simulink model "CRH2forBenchmark_Copy"  (R2014a)
settings: Solver=ode3  StartTime=0.0  StopTime=1  FixedStep=1e-5  RelTol=1e-3
PostLoadFcn:
  | , if any(exist('dsrtsu_mdlpostloadfcn', 'file') == [2, 3, 6]), try dsrtsu_mdlpostloadfcn('Execute', bdroot); catch fprintf('Error in PostLoadFcn (dsrtsu_mdlpostloadfcn) for model "%s":\n %s\n', bdroot, lasterr); end, end,
values from neighbouring files (symbols this model uses):
  Cd = 0.016    [CRH2forBenchmark.mat]
  Lm = 0.032848    [CRH2forBenchmark.mat]
  Ln = 0.002    [CRH2forBenchmark.mat]
  Lr = 0.034142    [CRH2forBenchmark.mat]
  Ls = 0.0342654    [CRH2forBenchmark.mat]
  np = 2    [CRH2forBenchmark.mat]
  Rd = 6000    [CRH2forBenchmark.mat]
  Rn = 0.2    [CRH2forBenchmark.mat]
  Rr = 0.146    [CRH2forBenchmark.mat]
  Rs = 0.144    [CRH2forBenchmark.mat]
  ts = 1e-05    [CRH2forBenchmark.mat]
undefined symbols (not defined in the file): J, KIM, KIT, KPM, KPT, phir, Ts, Vge
libraries: simulink x20
(part 4 of 5)

== system CRH2forBenchmark_Copy/ConverterF/Rectifier/RecSubF/SABF ==
  SA : Inport
  SB : Inport  Port=2
  SABF_sfcn : S-Function  FunctionName=SABF_sf  SFunctionModules=""  EnableBusSupport=off  mask{rtw_sf_name=SABF_sf, showVar=off}
      mask prompts: rtw_sf_name "Simulink:masks:GenSFuncName_MP"; showVar "Simulink:masks:GenSFuncShowModuleList_MP"
      mask help: Simulink:masks:GenSFuncDesc_MD
      mask init: same as CRH2forBenchmark_Copy/DCU1/DCU1_sfcn
      settings: CopyFcn=|
      | if ~strcmp(get_param(gcb,'Linkstatus'),'none') && ...
      | ~strcmp(get_param(gcb,'Linkstatus'),'implicit')
      |   set_param(gcb,'LinkStatus','none');
      | end
      mask Help: eval('feval(''rtwprivate'',''rtwhelpview'',''rtw_sfcn_block'')');
      mask Display:
      | port_label('input',1,'SA');
      | port_label('input',2,'SB');
      | port_label('output',1,'P');
      | port_label('output',2,'O');
      | port_label('output',3,'N');
  __InputSSForSFun__ : Subsystem
  __OutputSSForSFun__ : Subsystem
  P : Outport
  O : Outport  Port=2
  N : Outport  Port=3
  wires:
  SA/1 -> __InputSSForSFun__/1(SA)
  SB/1 -> __InputSSForSFun__/2(SB)
  __InputSSForSFun__/1(__UniqueOutportName__1__) -> SABF_sfcn/1
  __InputSSForSFun__/2(__UniqueOutportName__2__) -> SABF_sfcn/2
  SABF_sfcn/1 -> __OutputSSForSFun__/1(__UniqueInportName__1__)
  SABF_sfcn/2 -> __OutputSSForSFun__/2(__UniqueInportName__2__)
  SABF_sfcn/3 -> __OutputSSForSFun__/3(__UniqueInportName__3__)
  __OutputSSForSFun__/1(P) -> P/1
  __OutputSSForSFun__/2(O) -> O/1
  __OutputSSForSFun__/3(N) -> N/1

== system CRH2forBenchmark_Copy/ConverterF/Rectifier/RecSubF/SAF ==
  Ta1 : Inport
  Ta2 : Inport  Port=2
  Ta3 : Inport  Port=3
  Ta4 : Inport  Port=4
  In : Inport  Port=5
  SAF_sfcn : S-Function  FunctionName=SAF_sf  SFunctionModules=""  EnableBusSupport=off  mask{rtw_sf_name=SAF_sf, showVar=off}
      mask prompts: rtw_sf_name "Simulink:masks:GenSFuncName_MP"; showVar "Simulink:masks:GenSFuncShowModuleList_MP"
      mask help: Simulink:masks:GenSFuncDesc_MD
      mask init: same as CRH2forBenchmark_Copy/DCU1/DCU1_sfcn
      settings: CopyFcn=|
      | if ~strcmp(get_param(gcb,'Linkstatus'),'none') && ...
      | ~strcmp(get_param(gcb,'Linkstatus'),'implicit')
      |   set_param(gcb,'LinkStatus','none');
      | end
      mask Help: eval('feval(''rtwprivate'',''rtwhelpview'',''rtw_sfcn_block'')');
      mask Display:
      | port_label('input',1,'Ta1');
      | port_label('input',2,'Ta2');
      | port_label('input',3,'Ta3');
      | port_label('input',4,'Ta4');
      | port_label('input',5,'In');
      | port_label('output',1,'SA');
  __InputSSForSFun__ : Subsystem
  __OutputSSForSFun__ : Subsystem
  SA : Outport
  wires:
  Ta1/1 -> __InputSSForSFun__/1(Ta1)
  Ta2/1 -> __InputSSForSFun__/2(Ta2)
  Ta3/1 -> __InputSSForSFun__/3(Ta3)
  Ta4/1 -> __InputSSForSFun__/4(Ta4)
  In/1 -> __InputSSForSFun__/5(In)
  __InputSSForSFun__/1(__UniqueOutportName__1__) -> SAF_sfcn/1
  __InputSSForSFun__/2(__UniqueOutportName__2__) -> SAF_sfcn/2
  __InputSSForSFun__/3(__UniqueOutportName__3__) -> SAF_sfcn/3
  __InputSSForSFun__/4(__UniqueOutportName__4__) -> SAF_sfcn/4
  __InputSSForSFun__/5(__UniqueOutportName__5__) -> SAF_sfcn/5
  SAF_sfcn/1 -> __OutputSSForSFun__/1(__UniqueInportName__1__)
  __OutputSSForSFun__/1(SA) -> SA/1

== system CRH2forBenchmark_Copy/ConverterF/Rectifier/RecSubF/SBF ==
  Tb1 : Inport
  Tb2 : Inport  Port=2
  Tb3 : Inport  Port=3
  Tb4 : Inport  Port=4
  In : Inport  Port=5
  SBF_sfcn : S-Function  FunctionName=SBF_sf  SFunctionModules=""  EnableBusSupport=off  mask{rtw_sf_name=SBF_sf, showVar=off}
      mask prompts: rtw_sf_name "Simulink:masks:GenSFuncName_MP"; showVar "Simulink:masks:GenSFuncShowModuleList_MP"
      mask help: Simulink:masks:GenSFuncDesc_MD
      mask init: same as CRH2forBenchmark_Copy/DCU1/DCU1_sfcn
      settings: CopyFcn=|
      | if ~strcmp(get_param(gcb,'Linkstatus'),'none') && ...
      | ~strcmp(get_param(gcb,'Linkstatus'),'implicit')
      |   set_param(gcb,'LinkStatus','none');
      | end
      mask Help: eval('feval(''rtwprivate'',''rtwhelpview'',''rtw_sfcn_block'')');
      mask Display:
      | port_label('input',1,'Tb1');
      | port_label('input',2,'Tb2');
      | port_label('input',3,'Tb3');
      | port_label('input',4,'Tb4');
      | port_label('input',5,'In');
      | port_label('output',1,'SB');
  __InputSSForSFun__ : Subsystem
  __OutputSSForSFun__ : Subsystem
  SB : Outport
  wires:
  Tb1/1 -> __InputSSForSFun__/1(Tb1)
  Tb2/1 -> __InputSSForSFun__/2(Tb2)
  Tb3/1 -> __InputSSForSFun__/3(Tb3)
  Tb4/1 -> __InputSSForSFun__/4(Tb4)
  In/1 -> __InputSSForSFun__/5(In)
  __InputSSForSFun__/1(__UniqueOutportName__1__) -> SBF_sfcn/1
  __InputSSForSFun__/2(__UniqueOutportName__2__) -> SBF_sfcn/2
  __InputSSForSFun__/3(__UniqueOutportName__3__) -> SBF_sfcn/3
  __InputSSForSFun__/4(__UniqueOutportName__4__) -> SBF_sfcn/4
  __InputSSForSFun__/5(__UniqueOutportName__5__) -> SBF_sfcn/5
  SBF_sfcn/1 -> __OutputSSForSFun__/1(__UniqueInportName__1__)
  __OutputSSForSFun__/1(SB) -> SB/1

== system CRH2forBenchmark_Copy/ConverterN/Rectifier/RecSubN/RecSubSubN ==
  In1 : Inport
  In2 : Inport  Port=2
  In3 : Inport  Port=3
  In4 : Inport  Port=4
  In5 : Inport  Port=5
  In6 : Inport  Port=6
  RecSubSubN_sfcn : S-Function  FunctionName=RecSubSubN_sf  SFunctionModules=""  EnableBusSupport=off  mask{rtw_sf_name=RecSubSubN_sf, showVar=off}
      mask prompts: rtw_sf_name "Simulink:masks:GenSFuncName_MP"; showVar "Simulink:masks:GenSFuncShowModuleList_MP"
      mask help: Simulink:masks:GenSFuncDesc_MD
      mask init: same as CRH2forBenchmark_Copy/DCU1/DCU1_sfcn
      settings: CopyFcn=|
      | if ~strcmp(get_param(gcb,'Linkstatus'),'none') && ...
      | ~strcmp(get_param(gcb,'Linkstatus'),'implicit')
      |   set_param(gcb,'LinkStatus','none');
      | end
      mask Help: eval('feval(''rtwprivate'',''rtwhelpview'',''rtw_sfcn_block'')');
      mask Display:
      | port_label('input',1,'In1');
      | port_label('input',2,'In2');
      | port_label('input',3,'In3');
      | port_label('input',4,'In4');
      | port_label('input',5,'In5');
      | port_label('input',6,'In6');
      | port_label('output',1,'Out1');
      | port_label('output',2,'Out2');
  __InputSSForSFun__ : Subsystem
  __OutputSSForSFun__ : Subsystem
  Out1 : Outport
  Out2 : Outport  Port=2
  wires:
  In1/1 -> __InputSSForSFun__/1(In1)
  In2/1 -> __InputSSForSFun__/2(In2)
  In3/1 -> __InputSSForSFun__/3(In3)
  In4/1 -> __InputSSForSFun__/4(In4)
  In5/1 -> __InputSSForSFun__/5(In5)
  In6/1 -> __InputSSForSFun__/6(In6)
  __InputSSForSFun__/1(__UniqueOutportName__1__) -> RecSubSubN_sfcn/1
  __InputSSForSFun__/2(__UniqueOutportName__2__) -> RecSubSubN_sfcn/2
  __InputSSForSFun__/3(__UniqueOutportName__3__) -> RecSubSubN_sfcn/3
  __InputSSForSFun__/4(__UniqueOutportName__4__) -> RecSubSubN_sfcn/4
  __InputSSForSFun__/5(__UniqueOutportName__5__) -> RecSubSubN_sfcn/5
  __InputSSForSFun__/6(__UniqueOutportName__6__) -> RecSubSubN_sfcn/6
  RecSubSubN_sfcn/1 -> __OutputSSForSFun__/1(__UniqueInportName__1__)
  RecSubSubN_sfcn/2 -> __OutputSSForSFun__/2(__UniqueInportName__2__)
  __OutputSSForSFun__/1(Out1) -> Out1/1
  __OutputSSForSFun__/2(Out2) -> Out2/1

== system CRH2forBenchmark_Copy/ConverterN/Rectifier/RecSubN/SABN ==
  SA : Inport
  SB : Inport  Port=2
  SABN_sfcn : S-Function  FunctionName=SABN_sf  SFunctionModules=""  EnableBusSupport=off  mask{rtw_sf_name=SABN_sf, showVar=off}
      mask prompts: rtw_sf_name "Simulink:masks:GenSFuncName_MP"; showVar "Simulink:masks:GenSFuncShowModuleList_MP"
      mask help: Simulink:masks:GenSFuncDesc_MD
      mask init: same as CRH2forBenchmark_Copy/DCU1/DCU1_sfcn
      settings: CopyFcn=|
      | if ~strcmp(get_param(gcb,'Linkstatus'),'none') && ...
      | ~strcmp(get_param(gcb,'Linkstatus'),'implicit')
      |   set_param(gcb,'LinkStatus','none');
      | end
      mask Help: eval('feval(''rtwprivate'',''rtwhelpview'',''rtw_sfcn_block'')');
      mask Display:
      | port_label('input',1,'SA');
      | port_label('input',2,'SB');
      | port_label('output',1,'P');
      | port_label('output',2,'O');
      | port_label('output',3,'N');
  __InputSSForSFun__ : Subsystem
  __OutputSSForSFun__ : Subsystem
  P : Outport
  O : Outport  Port=2
  N : Outport  Port=3
  wires:
  SA/1 -> __InputSSForSFun__/1(SA)
  SB/1 -> __InputSSForSFun__/2(SB)
  __InputSSForSFun__/1(__UniqueOutportName__1__) -> SABN_sfcn/1
  __InputSSForSFun__/2(__UniqueOutportName__2__) -> SABN_sfcn/2
  SABN_sfcn/1 -> __OutputSSForSFun__/1(__UniqueInportName__1__)
  SABN_sfcn/2 -> __OutputSSForSFun__/2(__UniqueInportName__2__)
  SABN_sfcn/3 -> __OutputSSForSFun__/3(__UniqueInportName__3__)
  __OutputSSForSFun__/1(P) -> P/1
  __OutputSSForSFun__/2(O) -> O/1
  __OutputSSForSFun__/3(N) -> N/1

== system CRH2forBenchmark_Copy/ConverterN/Rectifier/RecSubN/SAN ==
  Ta1 : Inport
  Ta2 : Inport  Port=2
  Ta3 : Inport  Port=3
  Ta4 : Inport  Port=4
  In : Inport  Port=5
  SAN_sfcn : S-Function  FunctionName=SAN_sf  SFunctionModules=""  EnableBusSupport=off  mask{rtw_sf_name=SAN_sf, showVar=off}
      mask prompts: rtw_sf_name "Simulink:masks:GenSFuncName_MP"; showVar "Simulink:masks:GenSFuncShowModuleList_MP"
      mask help: Simulink:masks:GenSFuncDesc_MD
      mask init: same as CRH2forBenchmark_Copy/DCU1/DCU1_sfcn
      settings: CopyFcn=|
      | if ~strcmp(get_param(gcb,'Linkstatus'),'none') && ...
      | ~strcmp(get_param(gcb,'Linkstatus'),'implicit')
      |   set_param(gcb,'LinkStatus','none');
      | end
      mask Help: eval('feval(''rtwprivate'',''rtwhelpview'',''rtw_sfcn_block'')');
      mask Display:
      | port_label('input',1,'Ta1');
      | port_label('input',2,'Ta2');
      | port_label('input',3,'Ta3');
      | port_label('input',4,'Ta4');
      | port_label('input',5,'In');
      | port_label('output',1,'SA');
  __InputSSForSFun__ : Subsystem
  __OutputSSForSFun__ : Subsystem
  SA : Outport
  wires:
  Ta1/1 -> __InputSSForSFun__/1(Ta1)
  Ta2/1 -> __InputSSForSFun__/2(Ta2)
  Ta3/1 -> __InputSSForSFun__/3(Ta3)
  Ta4/1 -> __InputSSForSFun__/4(Ta4)
  In/1 -> __InputSSForSFun__/5(In)
  __InputSSForSFun__/1(__UniqueOutportName__1__) -> SAN_sfcn/1
  __InputSSForSFun__/2(__UniqueOutportName__2__) -> SAN_sfcn/2
  __InputSSForSFun__/3(__UniqueOutportName__3__) -> SAN_sfcn/3
  __InputSSForSFun__/4(__UniqueOutportName__4__) -> SAN_sfcn/4
  __InputSSForSFun__/5(__UniqueOutportName__5__) -> SAN_sfcn/5
  SAN_sfcn/1 -> __OutputSSForSFun__/1(__UniqueInportName__1__)
  __OutputSSForSFun__/1(SA) -> SA/1

== system CRH2forBenchmark_Copy/ConverterN/Rectifier/RecSubN/SBN ==
  Tb1 : Inport
  Tb2 : Inport  Port=2
  Tb3 : Inport  Port=3
  Tb4 : Inport  Port=4
  In : Inport  Port=5
  SBN_sfcn : S-Function  FunctionName=SBN_sf  SFunctionModules=""  EnableBusSupport=off  mask{rtw_sf_name=SBN_sf, showVar=off}
      mask prompts: rtw_sf_name "Simulink:masks:GenSFuncName_MP"; showVar "Simulink:masks:GenSFuncShowModuleList_MP"
      mask help: Simulink:masks:GenSFuncDesc_MD
      mask init: same as CRH2forBenchmark_Copy/DCU1/DCU1_sfcn
      settings: CopyFcn=|
      | if ~strcmp(get_param(gcb,'Linkstatus'),'none') && ...
      | ~strcmp(get_param(gcb,'Linkstatus'),'implicit')
      |   set_param(gcb,'LinkStatus','none');
      | end
      mask Help: eval('feval(''rtwprivate'',''rtwhelpview'',''rtw_sfcn_block'')');
      mask Display:
      | port_label('input',1,'Tb1');
      | port_label('input',2,'Tb2');
      | port_label('input',3,'Tb3');
      | port_label('input',4,'Tb4');
      | port_label('input',5,'In');
      | port_label('output',1,'SB');
  __InputSSForSFun__ : Subsystem
  __OutputSSForSFun__ : Subsystem
  SB : Outport
  wires:
  Tb1/1 -> __InputSSForSFun__/1(Tb1)
  Tb2/1 -> __InputSSForSFun__/2(Tb2)
  Tb3/1 -> __InputSSForSFun__/3(Tb3)
  Tb4/1 -> __InputSSForSFun__/4(Tb4)
  In/1 -> __InputSSForSFun__/5(In)
  __InputSSForSFun__/1(__UniqueOutportName__1__) -> SBN_sfcn/1
  __InputSSForSFun__/2(__UniqueOutportName__2__) -> SBN_sfcn/2
  __InputSSForSFun__/3(__UniqueOutportName__3__) -> SBN_sfcn/3
  __InputSSForSFun__/4(__UniqueOutportName__4__) -> SBN_sfcn/4
  __InputSSForSFun__/5(__UniqueOutportName__5__) -> SBN_sfcn/5
  SBN_sfcn/1 -> __OutputSSForSFun__/1(__UniqueInportName__1__)
  __OutputSSForSFun__/1(SB) -> SB/1

== system CRH2forBenchmark_Copy/Machine model/Normal ModelF/MeasurementF/__InputSSForSFun__ ==
  isα : Inport
  isβ : Inport  Port=2
  irα : Inport  Port=3
  irβ : Inport  Port=4
  TL : Inport  Port=5
  __UniqueOutportName__1__ : Outport
  __UniqueOutportName__2__ : Outport  Port=2
  __UniqueOutportName__3__ : Outport  Port=3
  __UniqueOutportName__4__ : Outport  Port=4
  __UniqueOutportName__5__ : Outport  Port=5
  wires:
  isα/1 -> __UniqueOutportName__1__/1
  isβ/1 -> __UniqueOutportName__2__/1
  irα/1 -> __UniqueOutportName__3__/1
  irβ/1 -> __UniqueOutportName__4__/1
  TL/1 -> __UniqueOutportName__5__/1

== system CRH2forBenchmark_Copy/Machine model/Normal ModelF/MeasurementF/__OutputSSForSFun__ ==
  __UniqueInportName__1__ : Inport
  __UniqueInportName__2__ : Inport  Port=2
  __UniqueInportName__3__ : Inport  Port=3
  Te : Outport
  ω : Outport  Port=2
  Isabc : Outport  Port=3
  wires:
  __UniqueInportName__1__/1 -> Te/1
  __UniqueInportName__2__/1 -> ω/1
  __UniqueInportName__3__/1 -> Isabc/1

== system CRH2forBenchmark_Copy/Machine model/Normal ModelF/MotorSubsystem1F/MotorSubsystem1FSub ==
  note: 1/(Ls*Lr-Lm*Lm)
  ψrβ : Inport
  Usβ : Inport  Port=2
  Add : Sum  Inputs=+-
  Add1 : Sum  Inputs=-+
  Gain : Gain  Gain=Lm
  Gain1 : Gain  Gain=Lr
  Gain2 : Gain  Gain=1/(Ls*Lr-Lm*Lm)
  Gain3 : Gain  Gain=Rs
  Integrator : Integrator
  isβ : Outport
  ψsβ : Outport  Port=2
  wires:
  Gain3/1 -> Add1/1
  ψrβ/1 -> Gain/1
  Gain2/1 -> isβ/1, Gain3/1
  Gain/1 -> Add/2
  Usβ/1 -> Add1/2
  Gain1/1 -> Add/1
  Add1/1 -> Integrator/1
  Add/1 -> Gain2/1
  Integrator/1 -> ψsβ/1, Gain1/1

== system CRH2forBenchmark_Copy/Machine model/Normal ModelF/MotorSubsystem2F/MotorSubsystem2FSub ==
  ψsα : Inport
  ψrβ : Inport  Port=2
  ω : Inport  Port=3
  1/(Ls*Lr-Lm*Lm) : Gain  Gain=1/(Ls*Lr-Lm*Lm)
  Add : Sum  Inputs=+-
  Add1 : Sum  Inputs=--
  Gain : Gain  Gain=Lm
  Gain1 : Gain  Gain=Ls
  Gain3 : Gain  Gain=Rr
  Integrator : Integrator
  Product : Product
  irα : Outport
  ψrα : Outport  Port=2
  wires:
  Add1/1 -> Integrator/1
  ω/1 -> Product/1
  Product/1 -> Add1/2
  ψrβ/1 -> Product/2
  Gain/1 -> Add/2
  Integrator/1 -> ψrα/1, Gain1/1
  1/(Ls*Lr-Lm*Lm)/1 -> irα/1, Gain3/1
  Add/1 -> 1/(Ls*Lr-Lm*Lm)/1
  ψsα/1 -> Gain/1
  Gain1/1 -> Add/1
  Gain3/1 -> Add1/1

== system CRH2forBenchmark_Copy/Machine model/Normal ModelF/MotorSubsystem3F/MotorSubsystem3FSub ==
  ψsβ : Inport
  ψrα : Inport  Port=2
  ω : Inport  Port=3
  1/(Ls*Lr-Lm*Lm) : Gain  Gain=1/(Ls*Lr-Lm*Lm)
  Add : Sum  Inputs=+-
  Add1 : Sum  Inputs=-+
  Gain : Gain  Gain=Lm
  Gain1 : Gain  Gain=Ls
  Gain3 : Gain  Gain=Rr
  Integrator : Integrator
  Product : Product
  irβ : Outport
  ψrβ : Outport  Port=2
  wires:
  Add1/1 -> Integrator/1
  Add/1 -> 1/(Ls*Lr-Lm*Lm)/1
  ψrα/1 -> Product/2
  Gain3/1 -> Add1/1
  1/(Ls*Lr-Lm*Lm)/1 -> irβ/1, Gain3/1
  ψsβ/1 -> Gain/1
  Gain1/1 -> Add/1
  Gain/1 -> Add/2
  ω/1 -> Product/1
  Product/1 -> Add1/2
  Integrator/1 -> ψrβ/1, Gain1/1

== system CRH2forBenchmark_Copy/Machine model/Normal ModelF/MotorSubsystemF/MotorSubsystemFSub ==
  note: 1/(Ls*Lr-Lm*Lm)
  ψrα : Inport
  Usα : Inport  Port=2
  Add : Sum  Inputs=+-
  Add1 : Sum  Inputs=-+
  Gain : Gain  Gain=Lm
  Gain1 : Gain  Gain=Lr
  Gain2 : Gain  Gain=1/(Ls*Lr-Lm*Lm)
  Gain3 : Gain  Gain=Rs
  Integrator : Integrator
  isα : Outport
  ψsα : Outport  Port=2
  wires:
  Add1/1 -> Integrator/1
  Add/1 -> Gain2/1
  Integrator/1 -> ψsα/1, Gain1/1
  Gain2/1 -> isα/1, Gain3/1
  Usα/1 -> Add1/2
  Gain3/1 -> Add1/1
  Gain1/1 -> Add/1
  ψrα/1 -> Gain/1
  Gain/1 -> Add/2

== system CRH2forBenchmark_Copy/Machine model/Normal ModelF/r2sF/__InputSSForSFun__ ==
  Ua : Inport
  Ub : Inport  Port=2
  Uc : Inport  Port=3
  __UniqueOutportName__1__ : Outport
  __UniqueOutportName__2__ : Outport  Port=2
  __UniqueOutportName__3__ : Outport  Port=3
  wires:
  Ua/1 -> __UniqueOutportName__1__/1
  Ub/1 -> __UniqueOutportName__2__/1
  Uc/1 -> __UniqueOutportName__3__/1

== system CRH2forBenchmark_Copy/Machine model/Normal ModelF/r2sF/__OutputSSForSFun__ ==
  __UniqueInportName__1__ : Inport
  __UniqueInportName__2__ : Inport  Port=2
  Usα : Outport
  Usβ : Outport  Port=2
  wires:
  __UniqueInportName__1__/1 -> Usα/1
  __UniqueInportName__2__/1 -> Usβ/1

== system CRH2forBenchmark_Copy/Machine model1/Normal ModelN/MeasurementN/__InputSSForSFun__ ==
  isα : Inport
  isβ : Inport  Port=2
  irα : Inport  Port=3
  irβ : Inport  Port=4
  TL : Inport  Port=5
  __UniqueOutportName__1__ : Outport
  __UniqueOutportName__2__ : Outport  Port=2
  __UniqueOutportName__3__ : Outport  Port=3
  __UniqueOutportName__4__ : Outport  Port=4
  __UniqueOutportName__5__ : Outport  Port=5
  wires:
  isα/1 -> __UniqueOutportName__1__/1
  isβ/1 -> __UniqueOutportName__2__/1
  irα/1 -> __UniqueOutportName__3__/1
  irβ/1 -> __UniqueOutportName__4__/1
  TL/1 -> __UniqueOutportName__5__/1

== system CRH2forBenchmark_Copy/Machine model1/Normal ModelN/MeasurementN/__OutputSSForSFun__ ==
  __UniqueInportName__1__ : Inport
  __UniqueInportName__2__ : Inport  Port=2
  __UniqueInportName__3__ : Inport  Port=3
  Te : Outport
  ω : Outport  Port=2
  Isabc : Outport  Port=3
  wires:
  __UniqueInportName__1__/1 -> Te/1
  __UniqueInportName__2__/1 -> ω/1
  __UniqueInportName__3__/1 -> Isabc/1

== system CRH2forBenchmark_Copy/Machine model1/Normal ModelN/MotorSubsystem1N/MotorSubsystem1NSub ==
  note: 1/(Ls*Lr-Lm*Lm)
  ψrβ : Inport
  Usβ : Inport  Port=2
  Add : Sum  Inputs=+-
  Add1 : Sum  Inputs=-+
  Gain : Gain  Gain=Lm
  Gain1 : Gain  Gain=Lr
  Gain2 : Gain  Gain=1/(Ls*Lr-Lm*Lm)
  Gain3 : Gain  Gain=Rs
  Integrator : Integrator
  isβ : Outport
  ψsβ : Outport  Port=2
  wires:
  Gain3/1 -> Add1/1
  ψrβ/1 -> Gain/1
  Gain2/1 -> isβ/1, Gain3/1
  Gain/1 -> Add/2
  Usβ/1 -> Add1/2
  Gain1/1 -> Add/1
  Add1/1 -> Integrator/1
  Add/1 -> Gain2/1
  Integrator/1 -> ψsβ/1, Gain1/1

== system CRH2forBenchmark_Copy/Machine model1/Normal ModelN/MotorSubsystem2N/MotorSubsystem2NSub ==
  ψsα : Inport
  ψrβ : Inport  Port=2
  ω : Inport  Port=3
  1/(Ls*Lr-Lm*Lm) : Gain  Gain=1/(Ls*Lr-Lm*Lm)
  Add : Sum  Inputs=+-
  Add1 : Sum  Inputs=--
  Gain : Gain  Gain=Lm
  Gain1 : Gain  Gain=Ls
  Gain3 : Gain  Gain=Rr
  Integrator : Integrator
  Product : Product
  irα : Outport
  ψrα : Outport  Port=2
  wires:
  Add1/1 -> Integrator/1
  ω/1 -> Product/1
  Product/1 -> Add1/2
  ψrβ/1 -> Product/2
  Gain/1 -> Add/2
  Integrator/1 -> ψrα/1, Gain1/1
  1/(Ls*Lr-Lm*Lm)/1 -> irα/1, Gain3/1
  Add/1 -> 1/(Ls*Lr-Lm*Lm)/1
  ψsα/1 -> Gain/1
  Gain1/1 -> Add/1
  Gain3/1 -> Add1/1

== system CRH2forBenchmark_Copy/Machine model1/Normal ModelN/MotorSubsystem3N/MotorSubsystem3NSub ==
  ψsβ : Inport
  ψrα : Inport  Port=2
  ω : Inport  Port=3
  1/(Ls*Lr-Lm*Lm) : Gain  Gain=1/(Ls*Lr-Lm*Lm)
  Add : Sum  Inputs=+-
  Add1 : Sum  Inputs=-+
  Gain : Gain  Gain=Lm
  Gain1 : Gain  Gain=Ls
  Gain3 : Gain  Gain=Rr
  Integrator : Integrator
  Product : Product
  irβ : Outport
  ψrβ : Outport  Port=2
  wires:
  Add1/1 -> Integrator/1
  Add/1 -> 1/(Ls*Lr-Lm*Lm)/1
  ψrα/1 -> Product/2
  Gain3/1 -> Add1/1
  1/(Ls*Lr-Lm*Lm)/1 -> irβ/1, Gain3/1
  ψsβ/1 -> Gain/1
  Gain1/1 -> Add/1
  Gain/1 -> Add/2
  ω/1 -> Product/1
  Product/1 -> Add1/2
  Integrator/1 -> ψrβ/1, Gain1/1

== system CRH2forBenchmark_Copy/Machine model1/Normal ModelN/MotorSubsystemN/MotorSubsystemNSub ==
  note: 1/(Ls*Lr-Lm*Lm)
  ψrα : Inport
  Usα : Inport  Port=2
  Add : Sum  Inputs=+-
  Add1 : Sum  Inputs=-+
  Gain : Gain  Gain=Lm
  Gain1 : Gain  Gain=Lr
  Gain2 : Gain  Gain=1/(Ls*Lr-Lm*Lm)
  Gain3 : Gain  Gain=Rs
  Integrator : Integrator
  isα : Outport
  ψsα : Outport  Port=2
  wires:
  Add1/1 -> Integrator/1
  Add/1 -> Gain2/1
  Integrator/1 -> ψsα/1, Gain1/1
  Gain2/1 -> isα/1, Gain3/1
  Usα/1 -> Add1/2
  Gain3/1 -> Add1/1
  Gain1/1 -> Add/1
  ψrα/1 -> Gain/1
  Gain/1 -> Add/2

== system CRH2forBenchmark_Copy/Machine model1/Normal ModelN/r2sN/__InputSSForSFun__ ==
  Ua : Inport
  Ub : Inport  Port=2
  Uc : Inport  Port=3
  __UniqueOutportName__1__ : Outport
  __UniqueOutportName__2__ : Outport  Port=2
  __UniqueOutportName__3__ : Outport  Port=3
  wires:
  Ua/1 -> __UniqueOutportName__1__/1
  Ub/1 -> __UniqueOutportName__2__/1
  Uc/1 -> __UniqueOutportName__3__/1

== system CRH2forBenchmark_Copy/Machine model1/Normal ModelN/r2sN/__OutputSSForSFun__ ==
  __UniqueInportName__1__ : Inport
  __UniqueInportName__2__ : Inport  Port=2
  Usα : Outport
  Usβ : Outport  Port=2
  wires:
  __UniqueInportName__1__/1 -> Usα/1
  __UniqueInportName__2__/1 -> Usβ/1

== system CRH2forBenchmark_Copy/Benchmark/CFI1/Subsystem2/Subsystem/Fault-States ==
  In1 : Inport
  Constant1 : Constant  Value=ContantofPowerDevice(1,1)
  Constant2 : Constant  Value=ContantofPowerDevice(2,1)
  Constant3 : Constant  Value=ContantofPowerDevice(3,1)
  Multiport Switch1 : MultiPortSwitch  DiagnosticForDefault=None
  Out1 : Outport
  wires:
  Constant2/1 -> Multiport Switch1/3
  Constant3/1 -> Multiport Switch1/4
  Constant1/1 -> Multiport Switch1/2
  In1/1 -> Multiport Switch1/1
  Multiport Switch1/1 -> Out1/1

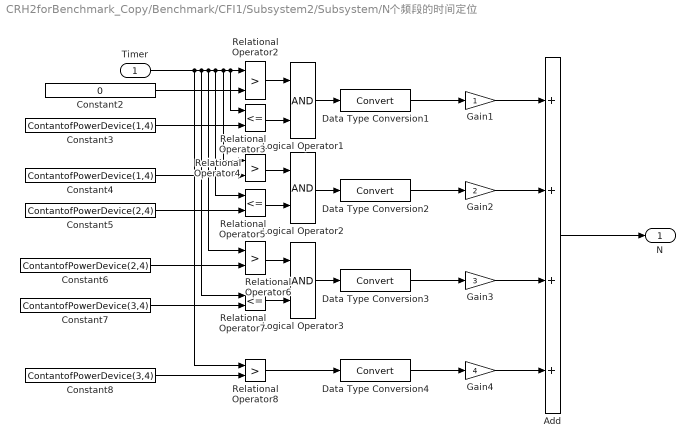
== system CRH2forBenchmark_Copy/Benchmark/CFI1/Subsystem2/Subsystem/N个频段的时间定位 ==
  Timer : Inport
  Add : Sum  Inputs=++++
  Constant2 : Constant  Value=0
  Constant3 : Constant  Value=ContantofPowerDevice(1,4)
  Constant4 : Constant  Value=ContantofPowerDevice(1,4)
  Constant5 : Constant  Value=ContantofPowerDevice(2,4)
  Constant6 : Constant  Value=ContantofPowerDevice(2,4)
  Constant7 : Constant  Value=ContantofPowerDevice(3,4)
  Constant8 : Constant  Value=ContantofPowerDevice(3,4)
  Data Type Conversion{1..4} (4 alike) : DataTypeConversion
  Gain1 : Gain
  Gain2 : Gain  Gain=2
  Gain3 : Gain  Gain=3
  Gain4 : Gain  Gain=4
  Logical Operator1 : Logic  AllPortsSameDT=off  OutDataTypeStr=boolean
  Logical Operator2 : Logic  AllPortsSameDT=off  OutDataTypeStr=boolean
  Logical Operator3 : Logic  AllPortsSameDT=off  OutDataTypeStr=boolean
  Relational Operator{2,4,6,8} (4 alike) : RelationalOperator  Operator=>  OutDataTypeStr=boolean
  Relational Operator3 : RelationalOperator  Operator=<=  OutDataTypeStr=boolean
  Relational Operator5 : RelationalOperator  Operator=<=  OutDataTypeStr=boolean
  Relational Operator7 : RelationalOperator  Operator=<=  OutDataTypeStr=boolean
  N : Outport
  wires:
  Gain4/1 -> Add/4
  Gain3/1 -> Add/3
  Gain2/1 -> Add/2
  Gain1/1 -> Add/1
  Add/1 -> N/1
  Constant8/1 -> Relational Operator8/2
  Constant7/1 -> Relational Operator7/2
  Constant6/1 -> Relational Operator6/2
  Constant5/1 -> Relational Operator5/2
  Constant4/1 -> Relational Operator4/2
  Constant3/1 -> Relational Operator3/2
  Constant2/1 -> Relational Operator2/2
  Timer/1 -> Relational Operator2/1, Relational Operator3/1, Relational Operator4/1, Relational Operator5/1, Relational Operator6/1, Relational Operator7/1, Relational Operator8/1
  Data Type Conversion4/1 -> Gain4/1
  Relational Operator8/1 -> Data Type Conversion4/1
  Data Type Conversion3/1 -> Gain3/1
  Logical Operator3/1 -> Data Type Conversion3/1
  Data Type Conversion2/1 -> Gain2/1
  Logical Operator2/1 -> Data Type Conversion2/1
  Data Type Conversion1/1 -> Gain1/1
  Logical Operator1/1 -> Data Type Conversion1/1
  Relational Operator7/1 -> Logical Operator3/2
  Relational Operator6/1 -> Logical Operator3/1
  Relational Operator5/1 -> Logical Operator2/2
  Relational Operator4/1 -> Logical Operator2/1
  Relational Operator3/1 -> Logical Operator1/2
  Relational Operator2/1 -> Logical Operator1/1

== system CRH2forBenchmark_Copy/Benchmark/CFI1/Subsystem2/Subsystem1/__InputSSForSFun__ ==
  Nomal : Inport
  Outside Signal1 : Inport  Port=2
  __UniqueOutportName__1__ : Outport
  __UniqueOutportName__2__ : Outport  Port=2
  __UniqueOutportName__3__ : Outport  Port=3
  __UniqueOutportName__4__ : Outport  Port=4
  wires:
  [PeriodicSignalsCFI1] -> __UniqueOutportName__4__/1
  [BandLimitedWhiteNoiseCFI1] -> __UniqueOutportName__3__/1
  Outside Signal1/1 -> __UniqueOutportName__2__/1
  Nomal/1 -> __UniqueOutportName__1__/1

== system CRH2forBenchmark_Copy/Benchmark/CFI1/Subsystem2/Subsystem1/__OutputSSForSFun__ ==
  __UniqueInportName__1__ : Inport
  Out : Outport
  wires:
  __UniqueInportName__1__/1 -> Out/1

== system CRH2forBenchmark_Copy/Benchmark/CFI2/Subsystem2/Subsystem/Fault-States ==
  In1 : Inport
  Constant1 : Constant  Value=ContantofPowerDevice(1,1)
  Constant2 : Constant  Value=ContantofPowerDevice(2,1)
  Constant3 : Constant  Value=ContantofPowerDevice(3,1)
  Multiport Switch1 : MultiPortSwitch  DiagnosticForDefault=None
  Out1 : Outport
  wires:
  Constant2/1 -> Multiport Switch1/3
  Constant3/1 -> Multiport Switch1/4
  Constant1/1 -> Multiport Switch1/2
  In1/1 -> Multiport Switch1/1
  Multiport Switch1/1 -> Out1/1

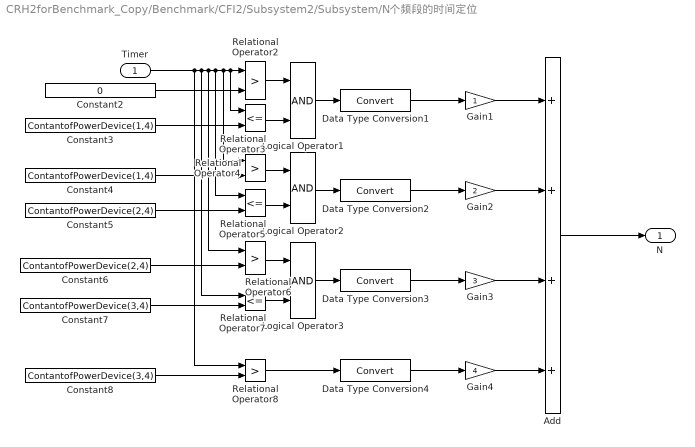
== system CRH2forBenchmark_Copy/Benchmark/CFI2/Subsystem2/Subsystem/N个频段的时间定位 ==
  Timer : Inport
  Add : Sum  Inputs=++++
  Constant2 : Constant  Value=0
  Constant3 : Constant  Value=ContantofPowerDevice(1,4)
  Constant4 : Constant  Value=ContantofPowerDevice(1,4)
  Constant5 : Constant  Value=ContantofPowerDevice(2,4)
  Constant6 : Constant  Value=ContantofPowerDevice(2,4)
  Constant7 : Constant  Value=ContantofPowerDevice(3,4)
  Constant8 : Constant  Value=ContantofPowerDevice(3,4)
  Data Type Conversion{1..4} (4 alike) : DataTypeConversion
  Gain1 : Gain
  Gain2 : Gain  Gain=2
  Gain3 : Gain  Gain=3
  Gain4 : Gain  Gain=4
  Logical Operator1 : Logic  AllPortsSameDT=off  OutDataTypeStr=boolean
  Logical Operator2 : Logic  AllPortsSameDT=off  OutDataTypeStr=boolean
  Logical Operator3 : Logic  AllPortsSameDT=off  OutDataTypeStr=boolean
  Relational Operator{2,4,6,8} (4 alike) : RelationalOperator  Operator=>  OutDataTypeStr=boolean
  Relational Operator3 : RelationalOperator  Operator=<=  OutDataTypeStr=boolean
  Relational Operator5 : RelationalOperator  Operator=<=  OutDataTypeStr=boolean
  Relational Operator7 : RelationalOperator  Operator=<=  OutDataTypeStr=boolean
  N : Outport
  wires:
  Gain4/1 -> Add/4
  Gain3/1 -> Add/3
  Gain2/1 -> Add/2
  Gain1/1 -> Add/1
  Add/1 -> N/1
  Constant8/1 -> Relational Operator8/2
  Constant7/1 -> Relational Operator7/2
  Constant6/1 -> Relational Operator6/2
  Constant5/1 -> Relational Operator5/2
  Constant4/1 -> Relational Operator4/2
  Constant3/1 -> Relational Operator3/2
  Constant2/1 -> Relational Operator2/2
  Timer/1 -> Relational Operator2/1, Relational Operator3/1, Relational Operator4/1, Relational Operator5/1, Relational Operator6/1, Relational Operator7/1, Relational Operator8/1
  Data Type Conversion4/1 -> Gain4/1
  Relational Operator8/1 -> Data Type Conversion4/1
  Data Type Conversion3/1 -> Gain3/1
  Logical Operator3/1 -> Data Type Conversion3/1
  Data Type Conversion2/1 -> Gain2/1
  Logical Operator2/1 -> Data Type Conversion2/1
  Data Type Conversion1/1 -> Gain1/1
  Logical Operator1/1 -> Data Type Conversion1/1
  Relational Operator7/1 -> Logical Operator3/2
  Relational Operator6/1 -> Logical Operator3/1
  Relational Operator5/1 -> Logical Operator2/2
  Relational Operator4/1 -> Logical Operator2/1
  Relational Operator3/1 -> Logical Operator1/2
  Relational Operator2/1 -> Logical Operator1/1

== system CRH2forBenchmark_Copy/Benchmark/CFI2/Subsystem2/Subsystem1/__InputSSForSFun__ ==
  Nomal : Inport
  Outside Signal1 : Inport  Port=2
  __UniqueOutportName__1__ : Outport
  __UniqueOutportName__2__ : Outport  Port=2
  __UniqueOutportName__3__ : Outport  Port=3
  __UniqueOutportName__4__ : Outport  Port=4
  wires:
  [PeriodicSignalsCFI2] -> __UniqueOutportName__4__/1
  [BandLimitedWhiteNoiseCFI2] -> __UniqueOutportName__3__/1
  Outside Signal1/1 -> __UniqueOutportName__2__/1
  Nomal/1 -> __UniqueOutportName__1__/1

== system CRH2forBenchmark_Copy/Benchmark/CFI2/Subsystem2/Subsystem1/__OutputSSForSFun__ ==
  __UniqueInportName__1__ : Inport
  Out : Outport
  wires:
  __UniqueInportName__1__/1 -> Out/1

== system CRH2forBenchmark_Copy/Benchmark/MFI1/MFI1/MFI /MFI1 ==
  Nomal : Inport
  Outside Signal1 : Inport  Port=2
  MFI_sfcn : S-Function  FunctionName=MFI_sf  Parameters=sfcnParam1, sfcnParam2, sfcnParam3, sfcnParam4, sfcnParam5, sfcnParam6, sfcnParam7, sfcnParam8, sfcnParam9  SFunctionModules=""  EnableBusSupport=off  mask{rtw_sf_name=MFI_sf, showVar=off, sfcnParam1=sfcnParam1, sfcnParam2=sfcnParam2, sfcnParam3=sfcnParam3, sfcnParam4=sfcnParam4, sfcnParam5=sfcnParam5, sfcnParam6=sfcnParam6, sfcnParam7=sfcnParam7, sfcnParam8=sfcnParam8, sfcnParam9=sfcnParam9}
      mask prompts: rtw_sf_name "Simulink:masks:GenSFuncName_MP"; showVar "Simulink:masks:GenSFuncShowModuleList_MP"; sfcnParam1 "AddMux:"; sfcnParam2 "BearingFP:"; sfcnParam3 "FS:"; sfcnParam4 "FaultInjectionTime:"; sfcnParam5 "FaultType:"; sfcnParam6 "NoiseSelec:"; sfcnParam7 "Severity1:"; sfcnParam8 "Severity2:"; sfcnParam9 "Severity3:"
      mask help: Simulink:masks:GenSFuncDesc_MD
      mask init: same as CRH2forBenchmark_Copy/DCU1/DCU1_sfcn
      settings: CopyFcn=|
      | if ~strcmp(get_param(gcb,'Linkstatus'),'none') && ...
      | ~strcmp(get_param(gcb,'Linkstatus'),'implicit')
      |   set_param(gcb,'LinkStatus','none');
      | end
      mask Help: eval('feval(''rtwprivate'',''rtwhelpview'',''rtw_sfcn_block'')');
      mask Display:
      | port_label('input',1,'Nomal');
      | port_label('input',2,'Outside Signal1');
      | port_label('input',3,'Inport1');
      | port_label('output',1,'Out');
  __InputSSForSFun__ : Subsystem
  __OutputSSForSFun__ : Subsystem
  Out : Outport
  wires:
  __OutputSSForSFun__/1(Out) -> Out/1
  MFI_sfcn/1 -> __OutputSSForSFun__/1(__UniqueInportName__1__)
  __InputSSForSFun__/3(__UniqueOutportName__3__) -> MFI_sfcn/3
  __InputSSForSFun__/2(__UniqueOutportName__2__) -> MFI_sfcn/2
  __InputSSForSFun__/1(__UniqueOutportName__1__) -> MFI_sfcn/1
  Outside Signal1/1 -> __InputSSForSFun__/2(Outside Signal1)
  Nomal/1 -> __InputSSForSFun__/1(Nomal)

== system CRH2forBenchmark_Copy/Benchmark/MFI1/MFI2/MFI /MFI1 ==
  Nomal : Inport
  Outside Signal1 : Inport  Port=2
  MFI_sfcn : S-Function  FunctionName=MFI_sf  Parameters=sfcnParam1, sfcnParam2, sfcnParam3, sfcnParam4, sfcnParam5, sfcnParam6, sfcnParam7, sfcnParam8, sfcnParam9  SFunctionModules=""  EnableBusSupport=off  mask{rtw_sf_name=MFI_sf, showVar=off, sfcnParam1=sfcnParam1, sfcnParam2=sfcnParam2, sfcnParam3=sfcnParam3, sfcnParam4=sfcnParam4, sfcnParam5=sfcnParam5, sfcnParam6=sfcnParam6, sfcnParam7=sfcnParam7, sfcnParam8=sfcnParam8, sfcnParam9=sfcnParam9}
      mask prompts: rtw_sf_name "Simulink:masks:GenSFuncName_MP"; showVar "Simulink:masks:GenSFuncShowModuleList_MP"; sfcnParam1 "AddMux:"; sfcnParam2 "BearingFP:"; sfcnParam3 "FS:"; sfcnParam4 "FaultInjectionTime:"; sfcnParam5 "FaultType:"; sfcnParam6 "NoiseSelec:"; sfcnParam7 "Severity1:"; sfcnParam8 "Severity2:"; sfcnParam9 "Severity3:"
      mask help: Simulink:masks:GenSFuncDesc_MD
      mask init: same as CRH2forBenchmark_Copy/DCU1/DCU1_sfcn
      settings: CopyFcn=|
      | if ~strcmp(get_param(gcb,'Linkstatus'),'none') && ...
      | ~strcmp(get_param(gcb,'Linkstatus'),'implicit')
      |   set_param(gcb,'LinkStatus','none');
      | end
      mask Help: eval('feval(''rtwprivate'',''rtwhelpview'',''rtw_sfcn_block'')');
      mask Display:
      | port_label('input',1,'Nomal');
      | port_label('input',2,'Outside Signal1');
      | port_label('input',3,'Inport1');
      | port_label('output',1,'Out');
  __InputSSForSFun__ : Subsystem
  __OutputSSForSFun__ : Subsystem
  Out : Outport
  wires:
  Nomal/1 -> __InputSSForSFun__/1(Nomal)
  Outside Signal1/1 -> __InputSSForSFun__/2(Outside Signal1)
  __InputSSForSFun__/1(__UniqueOutportName__1__) -> MFI_sfcn/1
  __InputSSForSFun__/2(__UniqueOutportName__2__) -> MFI_sfcn/2
  __InputSSForSFun__/3(__UniqueOutportName__3__) -> MFI_sfcn/3
  MFI_sfcn/1 -> __OutputSSForSFun__/1(__UniqueInportName__1__)
  __OutputSSForSFun__/1(Out) -> Out/1

== system CRH2forBenchmark_Copy/Benchmark/MFI1/MFI3/MFI /MFI1 ==
  Nomal : Inport
  Outside Signal1 : Inport  Port=2
  MFI_sfcn : S-Function  FunctionName=MFI_sf  Parameters=sfcnParam1, sfcnParam2, sfcnParam3, sfcnParam4, sfcnParam5, sfcnParam6, sfcnParam7, sfcnParam8, sfcnParam9  SFunctionModules=""  EnableBusSupport=off  mask{rtw_sf_name=MFI_sf, showVar=off, sfcnParam1=sfcnParam1, sfcnParam2=sfcnParam2, sfcnParam3=sfcnParam3, sfcnParam4=sfcnParam4, sfcnParam5=sfcnParam5, sfcnParam6=sfcnParam6, sfcnParam7=sfcnParam7, sfcnParam8=sfcnParam8, sfcnParam9=sfcnParam9}
      mask prompts: rtw_sf_name "Simulink:masks:GenSFuncName_MP"; showVar "Simulink:masks:GenSFuncShowModuleList_MP"; sfcnParam1 "AddMux:"; sfcnParam2 "BearingFP:"; sfcnParam3 "FS:"; sfcnParam4 "FaultInjectionTime:"; sfcnParam5 "FaultType:"; sfcnParam6 "NoiseSelec:"; sfcnParam7 "Severity1:"; sfcnParam8 "Severity2:"; sfcnParam9 "Severity3:"
      mask help: Simulink:masks:GenSFuncDesc_MD
      mask init: same as CRH2forBenchmark_Copy/DCU1/DCU1_sfcn
      settings: CopyFcn=|
      | if ~strcmp(get_param(gcb,'Linkstatus'),'none') && ...
      | ~strcmp(get_param(gcb,'Linkstatus'),'implicit')
      |   set_param(gcb,'LinkStatus','none');
      | end
      mask Help: eval('feval(''rtwprivate'',''rtwhelpview'',''rtw_sfcn_block'')');
      mask Display:
      | port_label('input',1,'Nomal');
      | port_label('input',2,'Outside Signal1');
      | port_label('input',3,'Inport1');
      | port_label('output',1,'Out');
  __InputSSForSFun__ : Subsystem
  __OutputSSForSFun__ : Subsystem
  Out : Outport
  wires:
  __OutputSSForSFun__/1(Out) -> Out/1
  MFI_sfcn/1 -> __OutputSSForSFun__/1(__UniqueInportName__1__)
  __InputSSForSFun__/3(__UniqueOutportName__3__) -> MFI_sfcn/3
  __InputSSForSFun__/2(__UniqueOutportName__2__) -> MFI_sfcn/2
  __InputSSForSFun__/1(__UniqueOutportName__1__) -> MFI_sfcn/1
  Outside Signal1/1 -> __InputSSForSFun__/2(Outside Signal1)
  Nomal/1 -> __InputSSForSFun__/1(Nomal)

== system CRH2forBenchmark_Copy/Benchmark/MFI1/MFI4/MFI /MFI1 ==
  Nomal : Inport
  Outside Signal1 : Inport  Port=2
  MFI_sfcn : S-Function  FunctionName=MFI_sf  Parameters=sfcnParam1, sfcnParam2, sfcnParam3, sfcnParam4, sfcnParam5, sfcnParam6, sfcnParam7, sfcnParam8, sfcnParam9  SFunctionModules=""  EnableBusSupport=off  mask{rtw_sf_name=MFI_sf, showVar=off, sfcnParam1=sfcnParam1, sfcnParam2=sfcnParam2, sfcnParam3=sfcnParam3, sfcnParam4=sfcnParam4, sfcnParam5=sfcnParam5, sfcnParam6=sfcnParam6, sfcnParam7=sfcnParam7, sfcnParam8=sfcnParam8, sfcnParam9=sfcnParam9}
      mask prompts: rtw_sf_name "Simulink:masks:GenSFuncName_MP"; showVar "Simulink:masks:GenSFuncShowModuleList_MP"; sfcnParam1 "AddMux:"; sfcnParam2 "BearingFP:"; sfcnParam3 "FS:"; sfcnParam4 "FaultInjectionTime:"; sfcnParam5 "FaultType:"; sfcnParam6 "NoiseSelec:"; sfcnParam7 "Severity1:"; sfcnParam8 "Severity2:"; sfcnParam9 "Severity3:"
      mask help: Simulink:masks:GenSFuncDesc_MD
      mask init: same as CRH2forBenchmark_Copy/DCU1/DCU1_sfcn
      settings: CopyFcn=|
      | if ~strcmp(get_param(gcb,'Linkstatus'),'none') && ...
      | ~strcmp(get_param(gcb,'Linkstatus'),'implicit')
      |   set_param(gcb,'LinkStatus','none');
      | end
      mask Help: eval('feval(''rtwprivate'',''rtwhelpview'',''rtw_sfcn_block'')');
      mask Display:
      | port_label('input',1,'Nomal');
      | port_label('input',2,'Outside Signal1');
      | port_label('input',3,'Inport1');
      | port_label('output',1,'Out');
  __InputSSForSFun__ : Subsystem
  __OutputSSForSFun__ : Subsystem
  Out : Outport
  wires:
  __OutputSSForSFun__/1(Out) -> Out/1
  MFI_sfcn/1 -> __OutputSSForSFun__/1(__UniqueInportName__1__)
  __InputSSForSFun__/3(__UniqueOutportName__3__) -> MFI_sfcn/3
  __InputSSForSFun__/2(__UniqueOutportName__2__) -> MFI_sfcn/2
  __InputSSForSFun__/1(__UniqueOutportName__1__) -> MFI_sfcn/1
  Outside Signal1/1 -> __InputSSForSFun__/2(Outside Signal1)
  Nomal/1 -> __InputSSForSFun__/1(Nomal)

== system CRH2forBenchmark_Copy/Benchmark/MFI1/MFI5/MFI /MFI1 ==
  Nomal : Inport
  Outside Signal1 : Inport  Port=2
  MFI_sfcn : S-Function  FunctionName=MFI_sf  Parameters=sfcnParam1, sfcnParam2, sfcnParam3, sfcnParam4, sfcnParam5, sfcnParam6, sfcnParam7, sfcnParam8, sfcnParam9  SFunctionModules=""  EnableBusSupport=off  mask{rtw_sf_name=MFI_sf, showVar=off, sfcnParam1=sfcnParam1, sfcnParam2=sfcnParam2, sfcnParam3=sfcnParam3, sfcnParam4=sfcnParam4, sfcnParam5=sfcnParam5, sfcnParam6=sfcnParam6, sfcnParam7=sfcnParam7, sfcnParam8=sfcnParam8, sfcnParam9=sfcnParam9}
      mask prompts: rtw_sf_name "Simulink:masks:GenSFuncName_MP"; showVar "Simulink:masks:GenSFuncShowModuleList_MP"; sfcnParam1 "AddMux:"; sfcnParam2 "BearingFP:"; sfcnParam3 "FS:"; sfcnParam4 "FaultInjectionTime:"; sfcnParam5 "FaultType:"; sfcnParam6 "NoiseSelec:"; sfcnParam7 "Severity1:"; sfcnParam8 "Severity2:"; sfcnParam9 "Severity3:"
      mask help: Simulink:masks:GenSFuncDesc_MD
      mask init: same as CRH2forBenchmark_Copy/DCU1/DCU1_sfcn
      settings: CopyFcn=|
      | if ~strcmp(get_param(gcb,'Linkstatus'),'none') && ...
      | ~strcmp(get_param(gcb,'Linkstatus'),'implicit')
      |   set_param(gcb,'LinkStatus','none');
      | end
      mask Help: eval('feval(''rtwprivate'',''rtwhelpview'',''rtw_sfcn_block'')');
      mask Display:
      | port_label('input',1,'Nomal');
      | port_label('input',2,'Outside Signal1');
      | port_label('input',3,'Inport1');
      | port_label('output',1,'Out');
  __InputSSForSFun__ : Subsystem
  __OutputSSForSFun__ : Subsystem
  Out : Outport
  wires:
  Nomal/1 -> __InputSSForSFun__/1(Nomal)
  Outside Signal1/1 -> __InputSSForSFun__/2(Outside Signal1)
  __InputSSForSFun__/1(__UniqueOutportName__1__) -> MFI_sfcn/1
  __InputSSForSFun__/2(__UniqueOutportName__2__) -> MFI_sfcn/2
  __InputSSForSFun__/3(__UniqueOutportName__3__) -> MFI_sfcn/3
  MFI_sfcn/1 -> __OutputSSForSFun__/1(__UniqueInportName__1__)
  __OutputSSForSFun__/1(Out) -> Out/1

== system CRH2forBenchmark_Copy/Benchmark/MFI1/MFI6/MFI /MFI1 ==
  Nomal : Inport
  Outside Signal1 : Inport  Port=2
  MFI_sfcn : S-Function  FunctionName=MFI_sf  Parameters=sfcnParam1, sfcnParam2, sfcnParam3, sfcnParam4, sfcnParam5, sfcnParam6, sfcnParam7, sfcnParam8, sfcnParam9  SFunctionModules=""  EnableBusSupport=off  mask{rtw_sf_name=MFI_sf, showVar=off, sfcnParam1=sfcnParam1, sfcnParam2=sfcnParam2, sfcnParam3=sfcnParam3, sfcnParam4=sfcnParam4, sfcnParam5=sfcnParam5, sfcnParam6=sfcnParam6, sfcnParam7=sfcnParam7, sfcnParam8=sfcnParam8, sfcnParam9=sfcnParam9}
      mask prompts: rtw_sf_name "Simulink:masks:GenSFuncName_MP"; showVar "Simulink:masks:GenSFuncShowModuleList_MP"; sfcnParam1 "AddMux:"; sfcnParam2 "BearingFP:"; sfcnParam3 "FS:"; sfcnParam4 "FaultInjectionTime:"; sfcnParam5 "FaultType:"; sfcnParam6 "NoiseSelec:"; sfcnParam7 "Severity1:"; sfcnParam8 "Severity2:"; sfcnParam9 "Severity3:"
      mask help: Simulink:masks:GenSFuncDesc_MD
      mask init: same as CRH2forBenchmark_Copy/DCU1/DCU1_sfcn
      settings: CopyFcn=|
      | if ~strcmp(get_param(gcb,'Linkstatus'),'none') && ...
      | ~strcmp(get_param(gcb,'Linkstatus'),'implicit')
      |   set_param(gcb,'LinkStatus','none');
      | end
      mask Help: eval('feval(''rtwprivate'',''rtwhelpview'',''rtw_sfcn_block'')');
      mask Display:
      | port_label('input',1,'Nomal');
      | port_label('input',2,'Outside Signal1');
      | port_label('input',3,'Inport1');
      | port_label('output',1,'Out');
  __InputSSForSFun__ : Subsystem
  __OutputSSForSFun__ : Subsystem
  Out : Outport
  wires:
  Nomal/1 -> __InputSSForSFun__/1(Nomal)
  Outside Signal1/1 -> __InputSSForSFun__/2(Outside Signal1)
  __InputSSForSFun__/1(__UniqueOutportName__1__) -> MFI_sfcn/1
  __InputSSForSFun__/2(__UniqueOutportName__2__) -> MFI_sfcn/2
  __InputSSForSFun__/3(__UniqueOutportName__3__) -> MFI_sfcn/3
  MFI_sfcn/1 -> __OutputSSForSFun__/1(__UniqueInportName__1__)
  __OutputSSForSFun__/1(Out) -> Out/1

== system CRH2forBenchmark_Copy/Benchmark/SFI1/Subsystem/SFI1/__InputSSForSFun__ ==
  Nomal : Inport
  Outside Signal : Inport  Port=2
  __UniqueOutportName__1__ : Outport
  __UniqueOutportName__2__ : Outport  Port=2
  __UniqueOutportName__3__ : Outport  Port=3
  __UniqueOutportName__4__ : Outport  Port=4
  wires:
  Nomal/1 -> __UniqueOutportName__1__/1
  Outside Signal/1 -> __UniqueOutportName__2__/1
  [BandLimitedWhiteNoiseSFI1] -> __UniqueOutportName__3__/1
  [PulseGeneratorSFI1] -> __UniqueOutportName__4__/1

== system CRH2forBenchmark_Copy/Benchmark/SFI1/Subsystem/SFI1/__OutputSSForSFun__ ==
  __UniqueInportName__1__ : Inport
  Out : Outport
  wires:
  __UniqueInportName__1__/1 -> Out/1

== system CRH2forBenchmark_Copy/Benchmark/SFI2/Subsystem/SFI1/__InputSSForSFun__ ==
  Nomal : Inport
  Outside Signal : Inport  Port=2
  __UniqueOutportName__1__ : Outport
  __UniqueOutportName__2__ : Outport  Port=2
  __UniqueOutportName__3__ : Outport  Port=3
  __UniqueOutportName__4__ : Outport  Port=4
  wires:
  Nomal/1 -> __UniqueOutportName__1__/1
  Outside Signal/1 -> __UniqueOutportName__2__/1
  [BandLimitedWhiteNoiseSFI2] -> __UniqueOutportName__3__/1
  [PulseGeneratorSFI2] -> __UniqueOutportName__4__/1

== system CRH2forBenchmark_Copy/Benchmark/SFI2/Subsystem/SFI1/__OutputSSForSFun__ ==
  __UniqueInportName__1__ : Inport
  Out : Outport
  wires:
  __UniqueInportName__1__/1 -> Out/1

== system CRH2forBenchmark_Copy/Benchmark/TFI1/TFI1Sub/Logic Operation/AddComp ==
  Add : Inport
  Constant : Constant  Value=Comp_ConV
  Constant1 : Constant  Value=Comp_ConV
  Max : simulink/Logic and Bit Operations/Compare To Constant  relop=<=  const=Comp_ConV  OutDataTypeStr=boolean
  Min : simulink/Logic and Bit Operations/Compare To Constant  relop=>=  const=Comp_ConV  OutDataTypeStr=boolean
  Switch : MultiPortSwitch  DataPortOrder=Zero-based contiguous  Inputs=2
  Switch2 : MultiPortSwitch  DataPortOrder=Zero-based contiguous  Inputs=2
  Out1 : Outport
  Out2 : Outport  Port=2
  wires:
  Switch2/1 -> Out2/1
  Constant1/1 -> Switch2/3
  Min/1 -> Switch/1
  Max/1 -> Switch2/1
  Constant/1 -> Switch/3
  Switch/1 -> Out1/1
  Add/1 -> Switch2/2, Min/1, Switch/2, Max/1

== system CRH2forBenchmark_Copy/Benchmark/TFI1/TFI1Sub/Logic Operation/MuxComp ==
  Mux : Inport
  Constant2 : Constant  Value=Comp_ConV
  Constant3 : Constant  Value=Comp_ConV
  Max1 : simulink/Logic and Bit Operations/Compare To Constant  relop=<=  const=Comp_ConV  OutDataTypeStr=boolean
  Min1 : simulink/Logic and Bit Operations/Compare To Constant  relop=>=  const=Comp_ConV  OutDataTypeStr=boolean
  Switch3 : MultiPortSwitch  DataPortOrder=Zero-based contiguous  Inputs=2
  Switch4 : MultiPortSwitch  DataPortOrder=Zero-based contiguous  Inputs=2
  Out1 : Outport
  Out2 : Outport  Port=2
  wires:
  Switch4/1 -> Out2/1
  Switch3/1 -> Out1/1
  Constant2/1 -> Switch3/3
  Max1/1 -> Switch4/1
  Constant3/1 -> Switch4/3
  Min1/1 -> Switch3/1
  Mux/1 -> Switch4/2, Min1/1, Switch3/2, Max1/1

== system CRH2forBenchmark_Copy/ConverterF/Rectifier/RecSubF/RecSubSubF/__InputSSForSFun__ ==
  In1 : Inport
  In2 : Inport  Port=2
  In3 : Inport  Port=3
  In4 : Inport  Port=4
  In5 : Inport  Port=5
  In6 : Inport  Port=6
  __UniqueOutportName__1__ : Outport
  __UniqueOutportName__2__ : Outport  Port=2
  __UniqueOutportName__3__ : Outport  Port=3
  __UniqueOutportName__4__ : Outport  Port=4
  __UniqueOutportName__5__ : Outport  Port=5
  __UniqueOutportName__6__ : Outport  Port=6
  wires:
  In1/1 -> __UniqueOutportName__1__/1
  In2/1 -> __UniqueOutportName__2__/1
  In3/1 -> __UniqueOutportName__3__/1
  In4/1 -> __UniqueOutportName__4__/1
  In5/1 -> __UniqueOutportName__5__/1
  In6/1 -> __UniqueOutportName__6__/1

== system CRH2forBenchmark_Copy/ConverterF/Rectifier/RecSubF/RecSubSubF/__OutputSSForSFun__ ==
  __UniqueInportName__1__ : Inport
  __UniqueInportName__2__ : Inport  Port=2
  Out1 : Outport
  Out2 : Outport  Port=2
  wires:
  __UniqueInportName__1__/1 -> Out1/1
  __UniqueInportName__2__/1 -> Out2/1

== system CRH2forBenchmark_Copy/ConverterF/Rectifier/RecSubF/SABF/__InputSSForSFun__ ==
  SA : Inport
  SB : Inport  Port=2
  __UniqueOutportName__1__ : Outport
  __UniqueOutportName__2__ : Outport  Port=2
  wires:
  SA/1 -> __UniqueOutportName__1__/1
  SB/1 -> __UniqueOutportName__2__/1

== system CRH2forBenchmark_Copy/ConverterF/Rectifier/RecSubF/SABF/__OutputSSForSFun__ ==
  __UniqueInportName__1__ : Inport
  __UniqueInportName__2__ : Inport  Port=2
  __UniqueInportName__3__ : Inport  Port=3
  P : Outport
  O : Outport  Port=2
  N : Outport  Port=3
  wires:
  __UniqueInportName__1__/1 -> P/1  "P"
  __UniqueInportName__2__/1 -> O/1  "O"
  __UniqueInportName__3__/1 -> N/1  "N"

== system CRH2forBenchmark_Copy/ConverterF/Rectifier/RecSubF/SAF/__InputSSForSFun__ ==
  Ta1 : Inport
  Ta2 : Inport  Port=2
  Ta3 : Inport  Port=3
  Ta4 : Inport  Port=4
  In : Inport  Port=5
  __UniqueOutportName__1__ : Outport
  __UniqueOutportName__2__ : Outport  Port=2
  __UniqueOutportName__3__ : Outport  Port=3
  __UniqueOutportName__4__ : Outport  Port=4
  __UniqueOutportName__5__ : Outport  Port=5
  wires:
  Ta1/1 -> __UniqueOutportName__1__/1
  Ta2/1 -> __UniqueOutportName__2__/1
  Ta3/1 -> __UniqueOutportName__3__/1
  Ta4/1 -> __UniqueOutportName__4__/1
  In/1 -> __UniqueOutportName__5__/1

== system CRH2forBenchmark_Copy/ConverterF/Rectifier/RecSubF/SAF/__OutputSSForSFun__ ==
  __UniqueInportName__1__ : Inport
  SA : Outport
  wires:
  __UniqueInportName__1__/1 -> SA/1

== system CRH2forBenchmark_Copy/ConverterF/Rectifier/RecSubF/SBF/__InputSSForSFun__ ==
  Tb1 : Inport
  Tb2 : Inport  Port=2
  Tb3 : Inport  Port=3
  Tb4 : Inport  Port=4
  In : Inport  Port=5
  __UniqueOutportName__1__ : Outport
  __UniqueOutportName__2__ : Outport  Port=2
  __UniqueOutportName__3__ : Outport  Port=3
  __UniqueOutportName__4__ : Outport  Port=4
  __UniqueOutportName__5__ : Outport  Port=5
  wires:
  Tb1/1 -> __UniqueOutportName__1__/1
  Tb2/1 -> __UniqueOutportName__2__/1
  Tb3/1 -> __UniqueOutportName__3__/1
  Tb4/1 -> __UniqueOutportName__4__/1
  In/1 -> __UniqueOutportName__5__/1

== system CRH2forBenchmark_Copy/ConverterF/Rectifier/RecSubF/SBF/__OutputSSForSFun__ ==
  __UniqueInportName__1__ : Inport
  SB : Outport
  wires:
  __UniqueInportName__1__/1 -> SB/1

== system CRH2forBenchmark_Copy/ConverterN/Rectifier/RecSubN/RecSubSubN/__InputSSForSFun__ ==
  In1 : Inport
  In2 : Inport  Port=2
  In3 : Inport  Port=3
  In4 : Inport  Port=4
  In5 : Inport  Port=5
  In6 : Inport  Port=6
  __UniqueOutportName__1__ : Outport
  __UniqueOutportName__2__ : Outport  Port=2
  __UniqueOutportName__3__ : Outport  Port=3
  __UniqueOutportName__4__ : Outport  Port=4
  __UniqueOutportName__5__ : Outport  Port=5
  __UniqueOutportName__6__ : Outport  Port=6
  wires:
  In1/1 -> __UniqueOutportName__1__/1
  In2/1 -> __UniqueOutportName__2__/1
  In3/1 -> __UniqueOutportName__3__/1
  In4/1 -> __UniqueOutportName__4__/1
  In5/1 -> __UniqueOutportName__5__/1
  In6/1 -> __UniqueOutportName__6__/1

== system CRH2forBenchmark_Copy/ConverterN/Rectifier/RecSubN/RecSubSubN/__OutputSSForSFun__ ==
  __UniqueInportName__1__ : Inport
  __UniqueInportName__2__ : Inport  Port=2
  Out1 : Outport
  Out2 : Outport  Port=2
  wires:
  __UniqueInportName__1__/1 -> Out1/1
  __UniqueInportName__2__/1 -> Out2/1

== system CRH2forBenchmark_Copy/ConverterN/Rectifier/RecSubN/SABN/__InputSSForSFun__ ==
  SA : Inport
  SB : Inport  Port=2
  __UniqueOutportName__1__ : Outport
  __UniqueOutportName__2__ : Outport  Port=2
  wires:
  SA/1 -> __UniqueOutportName__1__/1
  SB/1 -> __UniqueOutportName__2__/1

== system CRH2forBenchmark_Copy/ConverterN/Rectifier/RecSubN/SABN/__OutputSSForSFun__ ==
  __UniqueInportName__1__ : Inport
  __UniqueInportName__2__ : Inport  Port=2
  __UniqueInportName__3__ : Inport  Port=3
  P : Outport
  O : Outport  Port=2
  N : Outport  Port=3
  wires:
  __UniqueInportName__1__/1 -> P/1  "P"
  __UniqueInportName__2__/1 -> O/1  "O"
  __UniqueInportName__3__/1 -> N/1  "N"

== system CRH2forBenchmark_Copy/ConverterN/Rectifier/RecSubN/SAN/__InputSSForSFun__ ==
  Ta1 : Inport
  Ta2 : Inport  Port=2
  Ta3 : Inport  Port=3
  Ta4 : Inport  Port=4
  In : Inport  Port=5
  __UniqueOutportName__1__ : Outport
  __UniqueOutportName__2__ : Outport  Port=2
  __UniqueOutportName__3__ : Outport  Port=3
  __UniqueOutportName__4__ : Outport  Port=4
  __UniqueOutportName__5__ : Outport  Port=5
  wires:
  Ta1/1 -> __UniqueOutportName__1__/1
  Ta2/1 -> __UniqueOutportName__2__/1
  Ta3/1 -> __UniqueOutportName__3__/1
  Ta4/1 -> __UniqueOutportName__4__/1
  In/1 -> __UniqueOutportName__5__/1

== system CRH2forBenchmark_Copy/ConverterN/Rectifier/RecSubN/SAN/__OutputSSForSFun__ ==
  __UniqueInportName__1__ : Inport
  SA : Outport
  wires:
  __UniqueInportName__1__/1 -> SA/1
